simulink model "lab3_4_2-1"  (R2021b)
settings: Solver=VariableStepAuto  StartTime=0.0  StopTime=10.0  RelTol=1e-3
libraries: nonlinear_cart x1
settings Model: Creator=adanm  LastModifiedBy=Juho
settings SolverCC: AlgebraicLoopSolver=TrustRegion
settings DataIOCC: ReturnWorkspaceOutputs=off
settings DebuggingCC: SFMachineParentedDataDiag=warning  ArithmeticOperatorsInVariantConditions=warning
settings SFSimCC: CustomCodeUndefinedFunction=UseInterfaceOnly

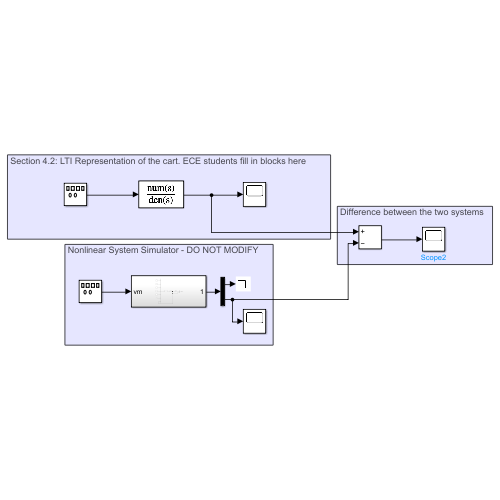
[thumbnail: Simulink's stored preview of the top-level diagram]
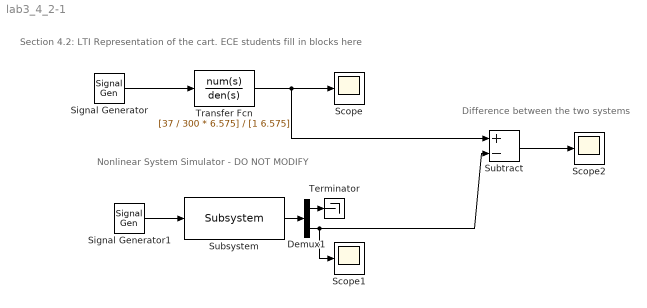
== system lab3_4_2-1 ==
  note: Section 4.2: LTI Representation of the cart. ECE students fill in blocks here
  note: Nonlinear System Simulator - DO NOT MODIFY
  note: Difference between the two systems
  Demux1 : Demux  Outputs=2
  Scope : Scope
  Scope1 : Scope
  Scope2 : Scope
  Signal Generator : SignalGenerator  WaveForm=square  Amplitude=1.5  Frequency=0.5
  Signal Generator1 : SignalGenerator  WaveForm=square  Amplitude=1.5  Frequency=0.5
  Subsystem : nonlinear_cart/Subsystem  SystemSampleTime=-1  VariantActivationTime=update diagram  Latency=0  AutoFrameSizeCalculation=off
  Subtract : Sum  Inputs=+-
  Terminator : Terminator
  Transfer Fcn : TransferFcn  Numerator=[37 / 300 * 6.575]  Denominator=[1 6.575]
  wires:
  Subsystem/1 -> Demux1/1
  Demux1/1 -> Terminator/1
  Transfer Fcn/1 -> Scope/1, Subtract/1
  Demux1/2 -> Subtract/2, Scope1/1
  Signal Generator1/1 -> Subsystem/1
  Signal Generator/1 -> Transfer Fcn/1
  Subtract/1 -> Scope2/1
